simulink model "sgMdl_IO611_CAN_HS_Loopback"  (R2024b)
settings: Solver=FixedStepAuto  StartTime=0.0  StopTime=inf  RelTol=1e-3  EnableMultiTasking=on
libraries: canmsglib x10, speedgoatlib_IO611 x3, speedgoatlib_CANLIN_OfA2 x2, slrealtimeutilitieslib x2, simulink x1, hdlsllib x1
Description:
  | IO611 - CAN HS Loopback
settings Model: ModifiedByFormat=Speedgoat  SimulationMode=external  ExtModeEnableFloating=off  ExtModeTrigDuration=100000  Creator=Speedgoat  LastModifiedBy=Speedgoat
settings SolverCC: ConcurrentTasks=on  AlgebraicLoopSolver=TrustRegion  PositivePriorityOrder=on  AutoInsertRateTranBlk=on  InsertRTBMode=Never (minimum delay)
settings DataIOCC: SaveFormat=StructureWithTime
settings OptimizationCC: BlockReduction=off  OptimizeBlockIOStorage=off  BufferReuse=off  ReuseModelBlockBuffer=off  GlobalBufferReuse=off  ExpressionFolding=off  LocalBlockOutputs=off  OptimizeDataStoreBuffers=off  BusAssignmentInplaceUpdate=off
settings DebuggingCC: InheritedTsInSrcMsg=none  TasksWithSamePriorityMsg=none  UnconnectedInputMsg=warning  UnconnectedOutputMsg=warning  UnconnectedLineMsg=warning
settings HardwareCC: ProdBitPerLong=64  ProdLongLongMode=on  ProdHWDeviceType=Intel->x86-64 (Linux 64)
settings ModelReferenceCC: EnableRefExpFcnMdlSchedulingChecks=on
settings SFSimCC: CustomCodeUndefinedFunction=UseInterfaceOnly
settings RTWCC: Description=Speedgoat Real-Time Target Machine  SystemTargetFile=speedgoat.tlc  TemplateMakefile=slrealtime_default_tmf  Toolchain=Simulink Real-Time Toolchain  BuildConfiguration=Faster Runs  TargetLang=C++  GPUComputeCapability=3.5  DLArmComputeVersion=19.05
settings SimulinkRealTimeTargetCC: SubcomponentCodeInterfacePackaging=Reusable function  InstructionSetFMA=off  LogToMDFFile=off  SLRTFileLogMaxRuns=10  UseGCCFastMath=on
settings ConfigComp: CovBoundaryAbsTol=1.0e-5

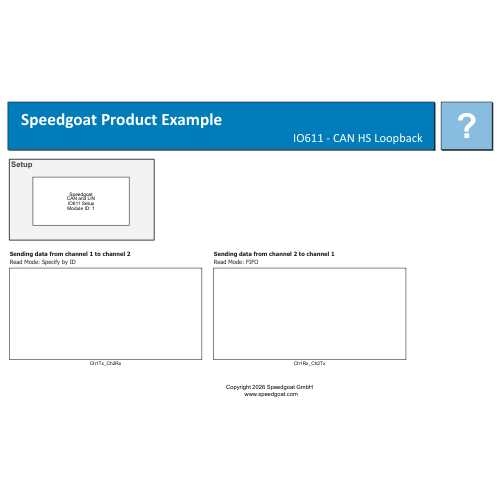
[thumbnail: Simulink's stored preview of the top-level diagram]
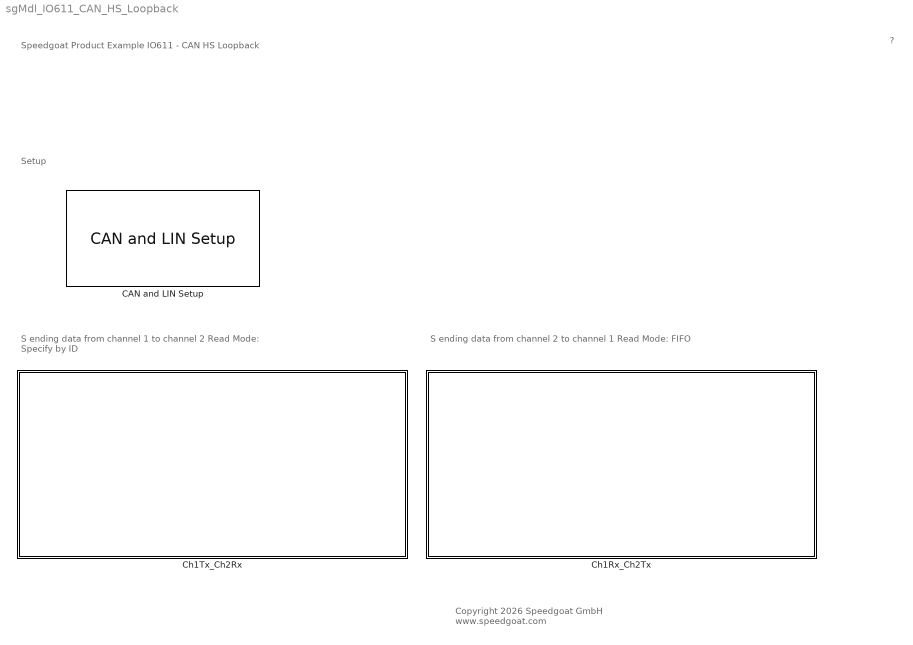
== system sgMdl_IO611_CAN_HS_Loopback ==
  note: S ending data from channel 2 to channel 1
      | Read Mode: FIFO
  note: S ending data from channel 1 to channel 2
      | Read Mode: Specify by ID
  note: Setup
  note: Speedgoat Product Example
      | IO611 - CAN HS Loopback
  note: ?
  note: Copyright 2026 Speedgoat GmbH
      |  www.speedgoat.com
  "CAN and LIN Setup " : speedgoatlib_IO611/CAN and LIN Setup   moduleInitValues="[611    1    1   -1   -1]"  id=1  moduleType=IO611  pciSlot=-1  canChn1=CAN (HS)  canChn2=CAN (HS)  canChn3=Disabled  canChn4=Disabled  linChn1=Disabled  linChn2=Disabled  canInitStructArray=[]  canTermStructArray=[]  canChn1InitValues="[2   2   1  31   8   2   1   5   2]"  arbBdrChn1=1.0 MBaud  arbManBdrChn1=[2,1,31,8]  fdBdrChn1=5.0 MBaud  fdManBdrChn1=[2,1,5,2]  canChn2InitValues="[2   2   1  31   8   2   1   5   2]"  arbBdrChn2=1.0 MBaud  arbManBdrChn2=[2,1,31,8]  fdBdrChn2=5.0 MBaud  fdManBdrChn2=[2,1,5,2]  canChn3InitValues="[1   2   1  31   8   2   1   5   2]"  arbBdrChn3=1.0 MBaud  arbManBdrChn3=[2,1,31,8]  fdBdrChn3=5.0 MBaud  fdManBdrChn3=[2,1,5,2]  canChn4InitValues="[1   2   1  31   8   2   1   5   2]"  arbBdrChn4=1.0 MBaud  arbManBdrChn4=[2,1,31,8]  fdBdrChn4=5.0 MBaud  fdManBdrChn4=[2,1,5,2]  bdrLIN1=19200  linChn1InitValues=[1 19800]  bdrLIN2=19200  linChn2InitValues=[1 19800]
      settings: SourceProductName=Simulink Real-Time: Speedgoat I/O Blockset
  Ch1Rx_Ch2Tx : Subsystem
  Ch1Tx_Ch2Rx : Subsystem

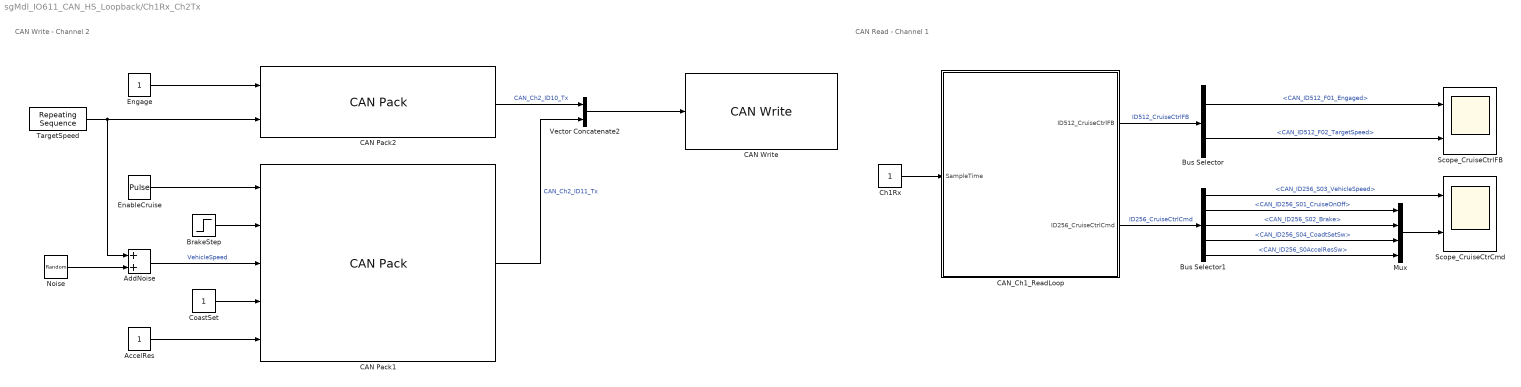
== system sgMdl_IO611_CAN_HS_Loopback/Ch1Rx_Ch2Tx ==
  note: CAN Read - Channel 1
  note: CAN Write - Channel 2
  AccelRes : Constant  SampleTime=-1
  AddNoise : Sum
  BrakeStep : Step  Time=6  SampleTime=0.005
  Bus Selector : BusSelector  OutputSignals=CAN_ID512_F01_Engaged,CAN_ID512_F02_TargetSpeed
  Bus Selector1 : BusSelector  OutputSignals=CAN_ID256_S03_VehicleSpeed,CAN_ID256_S01_CruiseOnOff,CAN_ID256_S02_Brake,CAN_ID256_S04_CoadtSetSw,CAN_ID256_S0AccelResSw
  CAN Pack1 : canmsglib/CAN Pack  MsgList=(none)  MsgName=CruiseCtrlCmd  MsgIDType=Standard (11-bit identifier)  MsgIdentifier=256  CANIDInput=off  MsgLength=2  Remote=off  ApplyMinMax=off  BusOutput=on  SignalInfo={ 'S01_CruiseOnOff', '0', '1', 'LE', 'unsigned', 'Standard', '0', '1', '0', '0', '1'; 'S02_Brake', '1', '1', 'LE', 'unsigned', 'Standard', '0', '1', '0', '0', '1'; 'S03_VehicleSpeed', '4', '8', 'LE', 'unsigned', 'Standard', '0', '1', '0', '0', '255'; 'S04_CoastSetSw', '2', '1', 'LE', 'unsigned', 'Standard', '0', '1', '0', '0', '1'; 'S05_AccelResSw', '3', '1', 'LE', 'unsigned', 'Standard', '0', '1', '0', '0', '1' }
      settings: DataFormat=manually specified signals
  CAN Pack2 : canmsglib/CAN Pack  MsgList=(none)  MsgName=CruiseCtrlFB  MsgIDType=Standard (11-bit identifier)  MsgIdentifier=512  CANIDInput=off  MsgLength=2  Remote=off  ApplyMinMax=off  BusOutput=on  SignalInfo={ 'F01_Engaged', '0', '1', 'LE', 'unsigned', 'Standard', '0', '1', '0', '0', '1'; 'F02_TargetSpeed', '1', '8', 'LE', 'unsigned', 'Standard', '0', '1', '0', '0', '255' }
      settings: DataFormat=manually specified signals
  "CAN Write " : speedgoatlib_CANLIN_OfA2/CAN Write   moduleType=IO611  id=1  channel=2  canType=CAN (HS)  useBusIn=on  numOfMsg=2  enableInput=off  enableStatusPort=off  initValues=[611 1 -1 1 1 1 0 2 0 1]  ts=-1
  CAN_Ch1_ReadLoop : Subsystem  TreatAsAtomicUnit=on
  Ch1Rx : Constant  SampleTime=0.005
  CoastSet : Constant  SampleTime=-1
  EnableCruise : DiscretePulseGenerator  Period=200  PulseWidth=100  SampleTime=0.005
  Engage : Constant  SampleTime=-1
  Mux : Mux
  Noise : RandomNumber
      settings: AttributesFormatString=|
      | Mean: %<Mean>
      | Variance: %<Variance>
  Scope_CruiseCtrCmd : Scope  NumInputPorts=2
  Scope_CruiseCtrlFB : Scope  NumInputPorts=2
  TargetSpeed : simulink/Sources/Repeating Sequence  rep_seq_t=[0 1 4 6 10]  rep_seq_y=[0 0 50 50 0]
  Vector Concatenate2 : Concatenate
  wires:
  CAN Pack2/1 -> Vector Concatenate2/1  "CAN_Ch2_ID10_Tx"
  AddNoise/1 -> CAN Pack1/3  "VehicleSpeed"
  Vector Concatenate2/1 -> "CAN Write "/1
  TargetSpeed/1 -> AddNoise/1, CAN Pack2/2
  AccelRes/1 -> CAN Pack1/5
  Bus Selector/1 -> Scope_CruiseCtrlFB/1  "<CAN_ID512_F01_Engaged>"
  CoastSet/1 -> CAN Pack1/4
  Noise/1 -> AddNoise/2
  CAN Pack1/1 -> Vector Concatenate2/2  "CAN_Ch2_ID11_Tx"
  Engage/1 -> CAN Pack2/1
  BrakeStep/1 -> CAN Pack1/2
  CAN_Ch1_ReadLoop/2(ID256_CruiseCtrlCmd) -> Bus Selector1/1  "ID256_CruiseCtrlCmd"
  EnableCruise/1 -> CAN Pack1/1
  CAN_Ch1_ReadLoop/1(ID512_CruiseCtrlFB) -> Bus Selector/1  "ID512_CruiseCtrlFB"
  Bus Selector1/1 -> Scope_CruiseCtrCmd/1  "<CAN_ID256_S03_VehicleSpeed>"
  Bus Selector/2 -> Scope_CruiseCtrlFB/2  "<CAN_ID512_F02_TargetSpeed>"
  Mux/1 -> Scope_CruiseCtrCmd/2
  Bus Selector1/5 -> Mux/4  "<CAN_ID256_S0AccelResSw>"
  Bus Selector1/3 -> Mux/2  "<CAN_ID256_S02_Brake>"
  Bus Selector1/4 -> Mux/3  "<CAN_ID256_S04_CoadtSetSw>"
  Bus Selector1/2 -> Mux/1  "<CAN_ID256_S01_CruiseOnOff>"
  Ch1Rx/1 -> CAN_Ch1_ReadLoop/1(SampleTime)

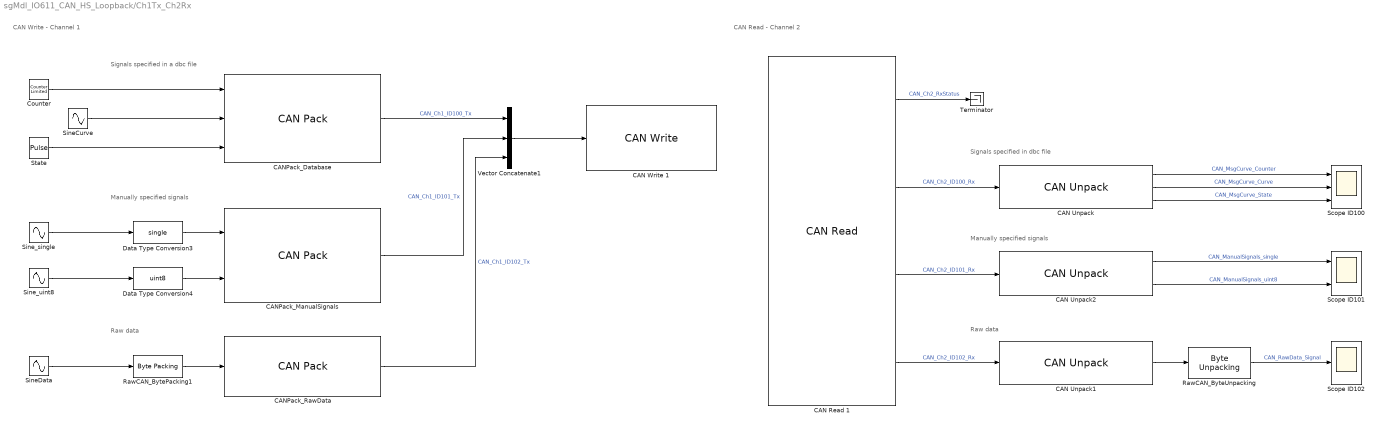
== system sgMdl_IO611_CAN_HS_Loopback/Ch1Tx_Ch2Rx ==
  note: Raw data
  note: Signals specified in dbc file
  note: Manually specified signals
  note: Signals specified in a dbc file
  note: Manually specified signals
  note: CAN Read - Channel 2
  note: CAN Write - Channel 1
  note: Raw data
  CAN Read 1 : speedgoatlib_IO611/CAN Read   moduleType=IO611  id=1  channel=2  canType=CAN (HS)  useBusOut=off  HasMulRead=Specify by IDs  MsgIDlist=[100:102]  isEFF=off  LabelInHex=off  enableInput=off  ts=-1  initValues=[611 1 -1 1 1 1 0 0 0 2 3 100 101 102]
      settings: SourceProductName=Simulink Real-Time: Speedgoat I/O Blockset
  CAN Unpack : canmsglib/CAN Unpack  CANdbFile=CANDatabase.dbc  MsgList=(none)  MsgName=MsgCurve  MsgIDType=Standard (11-bit identifier)  MsgIdentifier=100  MsgLength=4  SignalInfo={'Counter','16','7','LE','unsigned','Standard','0','1','0','-Inf','Inf';'Curve','0','16','LE','unsigned','Standard','0','0.1','0','0','6500';'State','23','1','LE','unsigned','Standard','0','1','0','0','1'}  IDPort=off  TimestampPort=off  ErrorPort=off  RemotePort=off  LengthPort=off  StatusPort=off  ApplyMinMax=off
      settings: DataFormat=CANdb specified signals
  CAN Unpack1 : canmsglib/CAN Unpack  MsgList=(none)  MsgName=Raw Data  MsgIDType=Standard (11-bit identifier)  MsgIdentifier=102  MsgLength=8  SignalInfo={ 'Counter', '16', '7', 'LE', 'unsigned', 'Standard', '0', '1', '0', '-Inf', 'Inf'; 'Curve', '0', '16', 'LE', 'unsigned', 'Standard', '0', '0.1', '0', '0', '6500'; 'State', '23', '1', 'LE', 'unsigned', 'Standard', '0', '1', '0', '0', '1' }  IDPort=off  TimestampPort=off  ErrorPort=off  RemotePort=off  LengthPort=off  StatusPort=off  ApplyMinMax=off
      settings: DataFormat=raw data
  CAN Unpack2 : canmsglib/CAN Unpack  MsgList=(none)  MsgName=Manual Signals  MsgIDType=Standard (11-bit identifier)  MsgIdentifier=101  MsgLength=5  SignalInfo={ 'single', '0', '32', 'LE', 'single', 'Standard', '0', '1', '0', '-Inf', 'Inf'; 'uint8', '32', '8', 'LE', 'unsigned', 'Standard', '0', '1', '0', '-Inf', 'Inf' }  IDPort=off  TimestampPort=off  ErrorPort=off  RemotePort=off  LengthPort=off  StatusPort=off  ApplyMinMax=off
  CAN Write 1 : speedgoatlib_IO611/CAN Write   moduleType=IO611  id=1  channel=1  canType=CAN (HS)  useBusIn=on  numOfMsg=3  enableInput=off  enableStatusPort=off  initValues=[611 1 -1 0 1 1 0 3 0 1]  ts=-1
      settings: SourceProductName=Simulink Real-Time: Speedgoat I/O Blockset
  CANPack_Database : canmsglib/CAN Pack  CANdbFile=CANDatabase.dbc  MsgList=MsgCurve  MsgName=MsgCurve  MsgIDType=Standard (11-bit identifier)  MsgIdentifier=100  CANIDInput=off  MsgLength=4  Remote=off  ApplyMinMax=off  BusOutput=on  SignalInfo={'Counter','16','7','LE','unsigned','Standard','0','1','0','-Inf','Inf';'Curve','0','16','LE','unsigned','Standard','0','0.1','0','0','6500';'State','23','1','LE','unsigned','Standard','0','1','0','0','1'}
      settings: DataFormat=CANdb specified signals
  CANPack_ManualSignals : canmsglib/CAN Pack  MsgList=(none)  MsgName=Manual Signals  MsgIDType=Standard (11-bit identifier)  MsgIdentifier=101  CANIDInput=off  MsgLength=5  Remote=off  ApplyMinMax=off  BusOutput=on  SignalInfo={ 'single', '0', '32', 'LE', 'single', 'Standard', '0', '1', '0', '-Inf', 'Inf'; 'uint8', '32', '8', 'LE', 'unsigned', 'Standard', '0', '1', '0', '-Inf', 'Inf' }
      settings: DataFormat=manually specified signals
  CANPack_RawData : canmsglib/CAN Pack  MsgList=(none)  MsgName=Raw Data  MsgIDType=Standard (11-bit identifier)  MsgIdentifier=102  CANIDInput=off  MsgLength=8  Remote=off  ApplyMinMax=off  BusOutput=on  SignalInfo={ 'Counter', '16', '7', 'LE', 'unsigned', 'Standard', '0', '1', '0', '-Inf', 'Inf'; 'Curve', '0', '16', 'LE', 'unsigned', 'Standard', '0', '0.1', '0', '0', '6500'; 'State', '23', '1', 'LE', 'unsigned', 'Standard', '0', '1', '0', '0', '1' }
      settings: DataFormat=raw data
  Counter : hdlsllib/Sources/Counter Limited  uplimit=127  tsamp=-1
  Data Type Conversion3 : DataTypeConversion  OutDataTypeStr=single  SaturateOnIntegerOverflow=off  RndMeth=Floor
  Data Type Conversion4 : DataTypeConversion  OutDataTypeStr=uint8  SaturateOnIntegerOverflow=off  RndMeth=Floor
  RawCAN_BytePacking1 : slrealtimeutilitieslib/Byte Packing  MaskPackedDataType=uint8  MaskUnpackedDataTypes={'double'}  MaskAlignment=1
  RawCAN_ByteUnpacking : slrealtimeutilitieslib/Byte Unpacking  MaskUnpackedDataTypes={'double'}  MaskUnpackedDataSizes={[1]}  MaskAlignment=1
  Scope ID100 : Scope  NumInputPorts=3
  Scope ID101 : Scope  NumInputPorts=2
  Scope ID102 : Scope
  SineCurve : Sin  Amplitude=30  Bias=50  Frequency=2*pi  SampleTime=0.005
  SineData : Sin  Amplitude=30  Bias=100  Frequency=2*pi  SampleTime=0.005
  Sine_single : Sin  Amplitude=30  Bias=100  Frequency=2*pi  SampleTime=0.005
  Sine_uint8 : Sin  Amplitude=30  Bias=50  Frequency=2*pi  SampleTime=0.005
  State : DiscretePulseGenerator  Period=200  PulseWidth=100  SampleTime=0.005
  Terminator : Terminator
  Vector Concatenate1 : Concatenate  NumInputs=3
  wires:
  RawCAN_ByteUnpacking/1 -> Scope ID102/1  "CAN_RawData_Signal"
  Sine_uint8/1 -> Data Type Conversion4/1
  CAN Unpack/3 -> Scope ID100/3  "CAN_MsgCurve_State"
  CAN Unpack/2 -> Scope ID100/2  "CAN_MsgCurve_Curve"
  Counter/1 -> CANPack_Database/1
  CANPack_Database/1 -> Vector Concatenate1/1  "CAN_Ch1_ID100_Tx"
  Sine_single/1 -> Data Type Conversion3/1
  Data Type Conversion3/1 -> CANPack_ManualSignals/1
  CAN Unpack2/2 -> Scope ID101/2  "CAN_ManualSignals_uint8"
  CAN Unpack2/1 -> Scope ID101/1  "CAN_ManualSignals_single"
  State/1 -> CANPack_Database/3
  CAN Read 1/4 -> CAN Unpack1/1  "CAN_Ch2_ID102_Rx"
  SineCurve/1 -> CANPack_Database/2
  CANPack_ManualSignals/1 -> Vector Concatenate1/2  "CAN_Ch1_ID101_Tx"
  CAN Read 1/1 -> Terminator/1  "CAN_Ch2_RxStatus"
  CAN Read 1/3 -> CAN Unpack2/1  "CAN_Ch2_ID101_Rx"
  CAN Read 1/2 -> CAN Unpack/1  "CAN_Ch2_ID100_Rx"
  Data Type Conversion4/1 -> CANPack_ManualSignals/2
  Vector Concatenate1/1 -> CAN Write 1/1
  CAN Unpack/1 -> Scope ID100/1  "CAN_MsgCurve_Counter"
  CAN Unpack1/1 -> RawCAN_ByteUnpacking/1
  RawCAN_BytePacking1/1 -> CANPack_RawData/1
  SineData/1 -> RawCAN_BytePacking1/1
  CANPack_RawData/1 -> Vector Concatenate1/3  "CAN_Ch1_ID102_Tx"

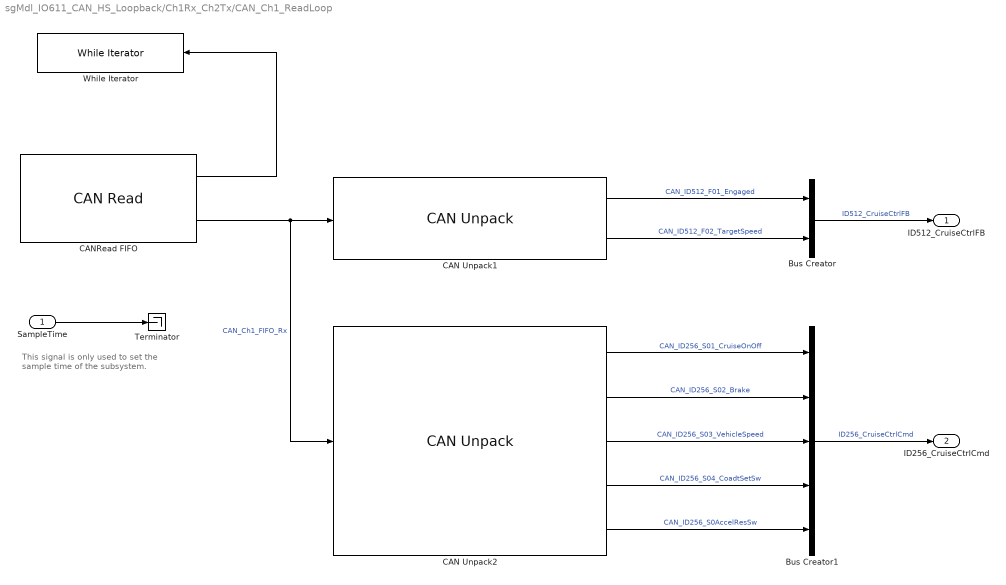
== system sgMdl_IO611_CAN_HS_Loopback/Ch1Rx_Ch2Tx/CAN_Ch1_ReadLoop ==
  note: This signal is only used to set the sample time of the subsystem.
  SampleTime : Inport
  Bus Creator : BusCreator  Inputs=2
  Bus Creator1 : BusCreator  Inputs=5
  CAN Unpack1 : canmsglib/CAN Unpack  MsgList=(none)  MsgName=CruiseCtrlFB  MsgIDType=Standard (11-bit identifier)  MsgIdentifier=512  MsgLength=2  SignalInfo={ 'F01_Engaged', '0', '1', 'LE', 'unsigned', 'Standard', '0', '1', '0', '0', '1'; 'F02_TargetSpeed', '1', '8', 'LE', 'unsigned', 'Standard', '0', '1', '0', '0', '255' }  IDPort=off  TimestampPort=off  ErrorPort=off  RemotePort=off  LengthPort=off  StatusPort=off  ApplyMinMax=off
  CAN Unpack2 : canmsglib/CAN Unpack  MsgList=(none)  MsgName=CruiseCtrlCmd  MsgIDType=Standard (11-bit identifier)  MsgIdentifier=256  MsgLength=2  SignalInfo={ 'S01_CruiseOnOff', '0', '1', 'LE', 'unsigned', 'Standard', '0', '1', '0', '0', '1'; 'S02_Brake', '1', '1', 'LE', 'unsigned', 'Standard', '0', '1', '0', '0', '1'; 'S03_VehicleSpeed', '4', '8', 'LE', 'unsigned', 'Standard', '0', '1', '0', '0', '255'; 'S04_CoastSetSw', '2', '1', 'LE', 'unsigned', 'Standard', '0', '1', '0', '0', '1'; 'S05_AccelResSw', '3', '1', 'LE', 'unsigned', 'Standard', '0', '1', '0', '0', '1' }  IDPort=off  TimestampPort=off  ErrorPort=off  RemotePort=off  LengthPort=off  StatusPort=off  ApplyMinMax=off
  CANRead FIFO : speedgoatlib_CANLIN_OfA2/CAN Read   moduleType=IO611  id=1  channel=1  canType=CAN (HS)  useBusOut=on  HasMulRead=Single Read from Buffer (FIFO)  MsgIDlist=[1,2]  isEFF=off  LabelInHex=on  enableInput=off  ts=-1  initValues=[611 1 -1 0 1 1 0 1 0 1 2 1 2]
  Terminator : Terminator
  While Iterator : WhileIterator  MaxIters=500  WhileBlockType=do-while
      settings: AttributesFormatString=|
      | ---
      | Max Numbers of iteration set to %<MaxIters>
      | This corresponds to the CAN HW buffer
  ID512_CruiseCtrlFB : Outport
  ID256_CruiseCtrlCmd : Outport  Port=2
  wires:
  CANRead FIFO/1 -> While Iterator/1
  CANRead FIFO/2 -> CAN Unpack2/1, CAN Unpack1/1  "CAN_Ch1_FIFO_Rx"
  CAN Unpack1/1 -> Bus Creator/1  "CAN_ID512_F01_Engaged"
  CAN Unpack1/2 -> Bus Creator/2  "CAN_ID512_F02_TargetSpeed"
  Bus Creator/1 -> ID512_CruiseCtrlFB/1  "ID512_CruiseCtrlFB"
  CAN Unpack2/1 -> Bus Creator1/1  "CAN_ID256_S01_CruiseOnOff"
  CAN Unpack2/2 -> Bus Creator1/2  "CAN_ID256_S02_Brake"
  CAN Unpack2/3 -> Bus Creator1/3  "CAN_ID256_S03_VehicleSpeed"
  CAN Unpack2/4 -> Bus Creator1/4  "CAN_ID256_S04_CoadtSetSw"
  CAN Unpack2/5 -> Bus Creator1/5  "CAN_ID256_S0AccelResSw"
  Bus Creator1/1 -> ID256_CruiseCtrlCmd/1  "ID256_CruiseCtrlCmd"
  SampleTime/1 -> Terminator/1
